simulink model "modelSS_temp2"  (R2021b)
settings: Solver=VariableStepAuto  StartTime=0.0  StopTime=1000000.0  RelTol=1e-3
undefined symbols (not defined in the file or in its folder): A, A_tilde, B, B_tilde, Bd, C, C_tilde, K, T_ambi_op
settings Model: Creator=martin  LastModifiedBy=kaspe

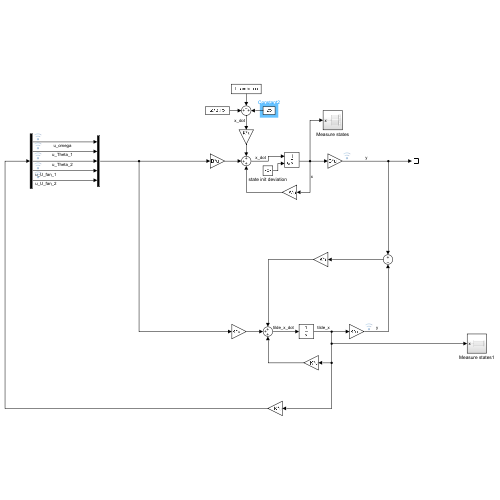
[thumbnail: Simulink's stored preview of the top-level diagram]
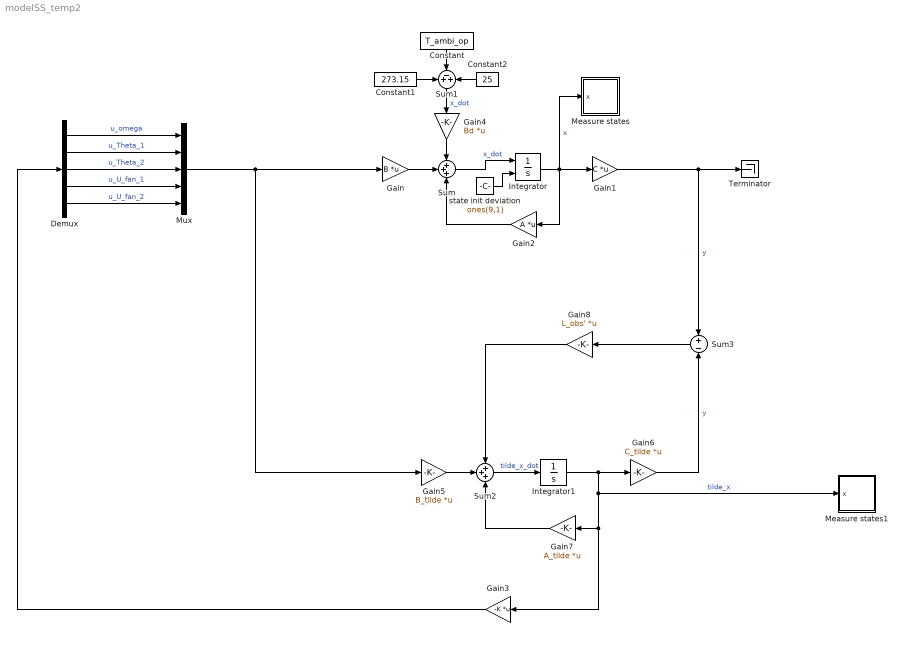
== system modelSS_temp2 ==
  Constant : Constant  Value=T_ambi_op
  Constant1 : Constant  Value=273.15  VectorParams1D=off
  Constant2 : Constant  Value=25  VectorParams1D=off
  Demux : Demux  Outputs=5
  Gain : Gain  Gain=B  Multiplication=Matrix(K*u)
  Gain1 : Gain  Gain=C  Multiplication=Matrix(K*u)
  Gain2 : Gain  Gain=A  Multiplication=Matrix(K*u)
  Gain3 : Gain  Gain=-K  Multiplication=Matrix(K*u)
  Gain4 : Gain  Gain=Bd  Multiplication=Matrix(K*u)
  Gain5 : Gain  Gain=B_tilde  Multiplication=Matrix(K*u)
  Gain6 : Gain  Gain=C_tilde  Multiplication=Matrix(K*u)
  Gain7 : Gain  Gain=A_tilde  Multiplication=Matrix(K*u)
  Gain8 : Gain  Gain=L_obs'  Multiplication=Matrix(K*u)
  Integrator : Integrator  InitialConditionSource=external
  Integrator1 : Integrator
  Measure states : Subsystem
  Measure states1 : Subsystem
  Mux : Mux  Inputs=5
  Sum : Sum  Inputs=+++
  Sum1 : Sum  Inputs=+-+
  Sum2 : Sum  Inputs=+++
  Sum3 : Sum  Inputs=+|-
  Terminator : Terminator
  state init deviation : Constant  Value=ones(9,1)
  wires:
  Sum/1 -> Integrator/1  "x_dot"
  Integrator/1 -> Gain2/1, Measure states/1(x), Gain1/1  "x"
  Gain2/1 -> Sum/3
  Gain/1 -> Sum/2
  Gain1/1 -> Sum3/1, Terminator/1  "y"
  Gain4/1 -> Sum/1
  Sum1/1 -> Gain4/1  "x_dot"
  Constant/1 -> Sum1/2
  Constant1/1 -> Sum1/1
  Demux/1 -> Mux/1  "u_omega"
  Demux/3 -> Mux/3  "u_Theta_2"
  Gain3/1 -> Demux/1
  Demux/2 -> Mux/2  "u_Theta_1"
  Demux/5 -> Mux/5  "u_U_fan_2"
  Demux/4 -> Mux/4  "u_U_fan_1"
  Constant2/1 -> Sum1/3
  Sum2/1 -> Integrator1/1  "tilde_x_dot"
  Mux/1 -> Gain/1, Gain5/1
  Gain5/1 -> Sum2/2
  Gain6/1 -> Sum3/2  "y"
  Gain7/1 -> Sum2/3
  Integrator1/1 -> Measure states1/1(x), Gain3/1, Gain7/1, Gain6/1  "tilde_x"
  Gain8/1 -> Sum2/1
  state init deviation/1 -> Integrator/2
  Sum3/1 -> Gain8/1

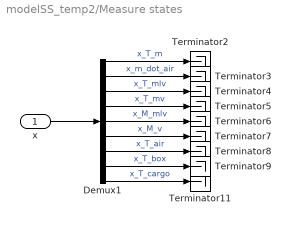
== system modelSS_temp2/Measure states ==
  x : Inport
  Demux1 : Demux  Outputs=9
  Terminator{2..9,11} (9 alike) : Terminator
  wires:
  Demux1/5 -> Terminator6/1  "x_M_mlv"
  Demux1/7 -> Terminator8/1  "x_T_air"
  Demux1/6 -> Terminator7/1  "x_M_v"
  Demux1/3 -> Terminator4/1  "x_T_mlv"
  Demux1/1 -> Terminator2/1  "x_T_m"
  Demux1/2 -> Terminator3/1  "x_m_dot_air"
  Demux1/4 -> Terminator5/1  "x_T_mv"
  Demux1/9 -> Terminator11/1  "x_T_cargo"
  Demux1/8 -> Terminator9/1  "x_T_box"
  x/1 -> Demux1/1

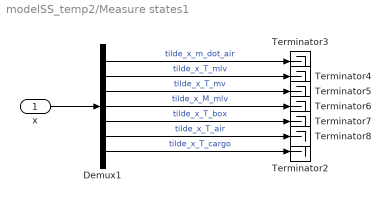
== system modelSS_temp2/Measure states1 ==
  x : Inport
  Demux1 : Demux  Outputs=7
  Terminator{2..8} (7 alike) : Terminator
  wires:
  Demux1/4 -> Terminator6/1  "tilde_x_M_mlv"
  Demux1/6 -> Terminator8/1  "tilde_x_T_air"
  Demux1/2 -> Terminator4/1  "tilde_x_T_mlv"
  Demux1/1 -> Terminator3/1  "tilde_x_m_dot_air"
  Demux1/3 -> Terminator5/1  "tilde_x_T_mv"
  Demux1/7 -> Terminator2/1  "tilde_x_T_cargo"
  Demux1/5 -> Terminator7/1  "tilde_x_T_box"
  x/1 -> Demux1/1
